simulink library "GOcontroll_Moduline_Target"  (R2023b)
settings: Solver=ode45  StartTime=0.0  StopTime=10.0  RelTol=1e-3  EnableMultiTasking=on
PreLoadFcn:
  | compile_gocontroll_mex;
values from neighbouring files (symbols this model uses):
  id = 2    [sfcn_UDPReceive.m]    (also in sfcn_UDPSend.m = 4)
undefined symbols (not defined in the file or in its folder): C_Cb1Pt10, Cb1Pt10_RAW_ERR_HIGH, Cb1Pt10_RAW_ERR_LOW, Cb1Pt10_SIG_ERR_HIGH, Cb1Pt10_SIG_ERR_LOW, Cb1Pt10_SIG_WAR_HIGH, Cb1Pt10_SIG_WAR_LOW, Pres_0_20_bar_500_4500_mv_inv, signal_x_RAW_ERR_HIGH, signal_x_RAW_ERR_LOW, signal_x_SIG_ERR_HIGH, signal_x_SIG_ERR_LOW, signal_x_SIG_WAR_HIGH, signal_x_SIG_WAR_LOW, signal_x_SPN, Valve1_ACTIVE_DUTY_CYCLE, Valve1_MAX_CURRENT, Valve1_MIN_CURRENT, Valve1_SPN
libraries: $bdroot x17, simulink x12, canmsglib x4
(part 5 of 5)

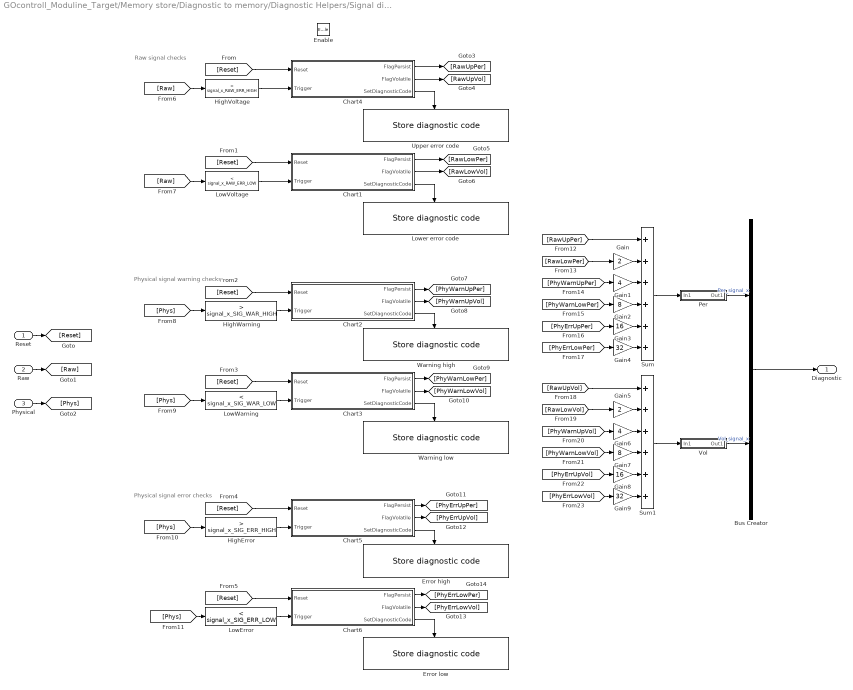
== system GOcontroll_Moduline_Target/Memory store/Diagnostic to memory/Diagnostic Helpers/Signal diagnostic ==
  note: Physical signal warning checks
  note: Raw signal checks
  note: Physical signal error checks
  Reset : Inport
  Raw : Inport  Port=2
  Physical : Inport  Port=3
  Enable : EnablePort
  Bus Creator : BusCreator  Inputs=2
  Chart1 : Stateflow chart  TreatAsAtomicUnit=on
  Chart2 : Stateflow chart  TreatAsAtomicUnit=on
  Chart3 : Stateflow chart  TreatAsAtomicUnit=on
  Chart4 : Stateflow chart  TreatAsAtomicUnit=on
  Chart5 : Stateflow chart  TreatAsAtomicUnit=on
  Chart6 : Stateflow chart  TreatAsAtomicUnit=on
  Error high : $bdroot/Memory store/Diagnostic to memory/Store diagnostic code  Tag=HANcoder_GOcontroll_Moduline_IV  spn=spn  fmi=(0) Data valid but above normal operational range, most severe level (3)  TriggerType=rising
  Error low : $bdroot/Memory store/Diagnostic to memory/Store diagnostic code  Tag=HANcoder_GOcontroll_Moduline_IV  spn=spn  fmi=(1) Data valid but below normal operational range, most severe level (3)  TriggerType=rising
  Gain : Gain  Gain=2
  Gain1 : Gain  Gain=4
  Gain2 : Gain  Gain=8
  Gain3 : Gain  Gain=16
  Gain4 : Gain  Gain=32
  Gain5 : Gain  Gain=2
  Gain6 : Gain  Gain=4
  Gain7 : Gain  Gain=8
  Gain8 : Gain  Gain=16
  Gain9 : Gain  Gain=32
  HighError : simulink/Logic and Bit Operations/Compare To Constant  relop=>  const=signal_x_SIG_ERR_HIGH  OutDataTypeStr=boolean
  HighVoltage : simulink/Logic and Bit Operations/Compare To Constant  relop=>  const=signal_x_RAW_ERR_HIGH  OutDataTypeStr=boolean
  HighWarning : simulink/Logic and Bit Operations/Compare To Constant  relop=>  const=signal_x_SIG_WAR_HIGH  OutDataTypeStr=boolean
  LowError : simulink/Logic and Bit Operations/Compare To Constant  relop=<  const=signal_x_SIG_ERR_LOW  OutDataTypeStr=boolean
  LowVoltage : simulink/Logic and Bit Operations/Compare To Constant  relop=<  const=signal_x_RAW_ERR_LOW  OutDataTypeStr=boolean
  LowWarning : simulink/Logic and Bit Operations/Compare To Constant  relop=<  const=signal_x_SIG_WAR_LOW  OutDataTypeStr=boolean
  Lower error code : $bdroot/Memory store/Diagnostic to memory/Store diagnostic code  Tag=HANcoder_GOcontroll_Moduline_IV  spn=spn  fmi=(4) Voltage below normal, or shorted to low source  TriggerType=rising
  Per : Subsystem
  Sum : Sum  Inputs=++++++  OutDataTypeStr=uint8
  Sum1 : Sum  Inputs=++++++  OutDataTypeStr=uint8
  Upper error code : $bdroot/Memory store/Diagnostic to memory/Store diagnostic code  Tag=HANcoder_GOcontroll_Moduline_IV  spn=spn  fmi=(3) Voltage above normal, or shorted to high source  TriggerType=rising
  Vol : Subsystem
  Warning high : $bdroot/Memory store/Diagnostic to memory/Store diagnostic code  Tag=HANcoder_GOcontroll_Moduline_IV  spn=spn  fmi=(15) Data valid but above normal range: least severe level (1)  TriggerType=rising
  Warning low : $bdroot/Memory store/Diagnostic to memory/Store diagnostic code  Tag=HANcoder_GOcontroll_Moduline_IV  spn=spn  fmi=(17) Data valid but below normal range: least severe level (1)  TriggerType=rising
  Diagnostic : Outport  OutputWhenDisabled=reset  InitialOutput=[0]
  wires:
  Chart4/3(SetDiagnosticCode) -> Upper error code/Trigger
  HighVoltage/1 -> Chart4/2(Trigger)
  LowVoltage/1 -> Chart1/2(Trigger)
  Chart1/3(SetDiagnosticCode) -> Lower error code/Trigger
  HighWarning/1 -> Chart2/2(Trigger)
  Chart2/3(SetDiagnosticCode) -> Warning high/Trigger
  LowWarning/1 -> Chart3/2(Trigger)
  Chart3/3(SetDiagnosticCode) -> Warning low/Trigger
  Chart6/3(SetDiagnosticCode) -> Error low/Trigger
  Chart5/3(SetDiagnosticCode) -> Error high/Trigger
  HighError/1 -> Chart5/2(Trigger)
  LowError/1 -> Chart6/2(Trigger)
  Reset/1 -> [Reset]
  [Reset] -> Chart4/1(Reset)
  [Reset] -> Chart1/1(Reset)
  [Reset] -> Chart2/1(Reset)
  [Reset] -> Chart3/1(Reset)
  [Reset] -> Chart5/1(Reset)
  [Reset] -> Chart6/1(Reset)
  Raw/1 -> [Raw]
  [Raw] -> HighVoltage/1
  [Raw] -> LowVoltage/1
  Physical/1 -> [Phys]
  [Phys] -> HighWarning/1
  [Phys] -> LowWarning/1
  [Phys] -> HighError/1
  [Phys] -> LowError/1
  Chart4/1(FlagPersist) -> [RawUpPer]
  Chart4/2(FlagVolatile) -> [RawUpVol]
  Chart1/1(FlagPersist) -> [RawLowPer]
  Chart1/2(FlagVolatile) -> [RawLowVol]
  Chart2/1(FlagPersist) -> [PhyWarnUpPer]
  Chart2/2(FlagVolatile) -> [PhyWarnUpVol]
  Chart3/1(FlagPersist) -> [PhyWarnLowPer]
  Chart3/2(FlagVolatile) -> [PhyWarnLowVol]
  Chart5/1(FlagPersist) -> [PhyErrUpPer]
  Chart5/2(FlagVolatile) -> [PhyErrUpVol]
  Chart6/1(FlagPersist) -> [PhyErrLowPer]
  Chart6/2(FlagVolatile) -> [PhyErrLowVol]
  [RawUpPer] -> Sum/1
  [RawLowPer] -> Gain/1
  Gain/1 -> Sum/2
  Gain1/1 -> Sum/3
  Gain4/1 -> Sum/6
  Gain3/1 -> Sum/5
  Gain2/1 -> Sum/4
  [PhyWarnUpPer] -> Gain1/1
  [PhyWarnLowPer] -> Gain2/1
  [PhyErrUpPer] -> Gain3/1
  [PhyErrLowPer] -> Gain4/1
  Sum/1 -> Per/1(In1)
  [RawUpVol] -> Sum1/1
  Gain9/1 -> Sum1/6
  Sum1/1 -> Vol/1(In1)
  Gain6/1 -> Sum1/3
  Gain5/1 -> Sum1/2
  Gain7/1 -> Sum1/4
  Gain8/1 -> Sum1/5
  [RawLowVol] -> Gain5/1
  [PhyWarnLowVol] -> Gain7/1
  [PhyWarnUpVol] -> Gain6/1
  [PhyErrUpVol] -> Gain8/1
  [PhyErrLowVol] -> Gain9/1
  Bus Creator/1 -> Diagnostic/1
  Vol/1(Out1) -> Bus Creator/2  "Vol_signal_x"
  Per/1(Out1) -> Bus Creator/1  "Per_signal_x"

== system GOcontroll_Moduline_Target/Network/UDP/UDP Example/Decode ==
  message : Inport
  message length : Inport  Port=2
  function : TriggerPort  TriggerType=function-call  VariantControl=(inherit)
  Compare To Constant : simulink/Logic and Bit Operations/Compare To Constant  relop===  const=5  OutDataTypeStr=boolean
  message len ok : Subsystem
  wires:
  message/1 -> message len ok/1(In1)
  message length/1 -> Compare To Constant/1
  Compare To Constant/1 -> message len ok/Enable

== system GOcontroll_Moduline_Target/Memory store/Diagnostic to memory/Diagnostic Helpers/Actuator diagnostic/Per ==
  In1 : Inport
  Out1 : Outport
  wires:
  In1/1 -> Out1/1

== system GOcontroll_Moduline_Target/Memory store/Diagnostic to memory/Diagnostic Helpers/Actuator diagnostic/Vol ==
  In1 : Inport
  Out1 : Outport
  wires:
  In1/1 -> Out1/1

== system GOcontroll_Moduline_Target/Memory store/Diagnostic to memory/Diagnostic Helpers/Signal diagnostic/Per ==
  In1 : Inport
  Out1 : Outport
  wires:
  In1/1 -> Out1/1

== system GOcontroll_Moduline_Target/Memory store/Diagnostic to memory/Diagnostic Helpers/Signal diagnostic/Vol ==
  In1 : Inport
  Out1 : Outport
  wires:
  In1/1 -> Out1/1

== system GOcontroll_Moduline_Target/Network/UDP/UDP Example/Decode/message len ok ==
  note: extract the data from bytes 1-4
  note: Check that the message ID in byte0 matches
  In1 : Inport
  Enable : EnablePort
  Compare To Constant1 : simulink/Logic and Bit Operations/Compare To Constant  relop===  const=0  OutDataTypeStr=boolean
  Selector : Selector  IndexMode=Zero-based  InputPortWidth=5  IndexOptions=Index vector (dialog)  Indices=[0]  OutputSizes=1
  Selector1 : Selector  IndexMode=Zero-based  InputPortWidth=5  IndexOptions=Starting index (dialog)  Indices=[1]  OutputSizes=4
  message id ok : Subsystem
  wires:
  Selector1/1 -> message id ok/1(In1)
  Selector/1 -> Compare To Constant1/1
  Compare To Constant1/1 -> message id ok/Enable
  In1/1 -> Selector/1, Selector1/1

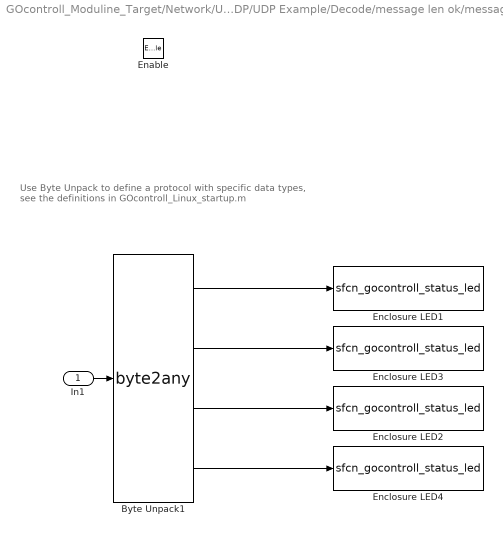
== system GOcontroll_Moduline_Target/Network/UDP/UDP Example/Decode/message len ok/message id ok ==
  note: Use Byte Unpack to define a protocol with
      | specific data types, see the definitions in
      | GOcontroll_Linux_startup.m
  In1 : Inport
  Enable : EnablePort
  Byte Unpack1 : S-Function  AncestorBlock=etargetslib/Byte Unpack  FunctionName=byte2any  Parameters=dimensionsout, datatypesout, byteAlign  SFunctionDeploymentMode=off  EnableBusSupport=off  mask(Byte Unpack){dimensions={1,1,1,1};, datatypes={'uint8','uint8','uint8','uint8'}, byteAlign=1}
      mask prompts: dimensions "Output port dimensions (cell array):"; datatypes "Output port data types (cell array):"; byteAlign "Byte alignment:"
      mask help: Unpack a binary byte vector to extract data. Insert after a UDP Recv block to break-up a UDP packet into its constituent data vectors.
      mask init:
      | [dimensionsout, datatypesout]= byteunpack_callback(dimensions, datatypes);
      mask Help: eval('linkfoundation.util.openBlockHelp(''etargetslibbyteunpack'')');
      mask TypeOptions byteAlign: 1 | 2 | 4 | 8
      mask Display:
      | color('blue');
      | text(0.95, 0.90, '', ...
      |                 'horizontalalignment', 'right');
      | color('black');
      | text(0.50, 0.12, 'Byte Unpack', ...
      |                 'horizontalAlignment','center');
  Enclosure LED1 : M-S-Function  Tag=HANcoder_TARGET_STM32_Olimexino  AncestorBlock=GOcontroll_Moduline_Target/Enclosure LED's/Enclosure LED  FunctionName=sfcn_gocontroll_status_led  Parameters=tsamp  mask(Enclosure LED's){tsamp=-1, led=1, color=Blue}
      mask prompts: tsamp "Sample time"
      mask help:
      | The Moduline controller is equipped with 4 RGB status LED's. To control them, simply configure the mask ( LED and color) and control them using uint8 values.
      |
      | Note: Moduline IV HW >= 3.02 has duty cycle controlled LED's. The intensity can be set from 0 (0%) to 255 (100%).
      |
      | LED: Select the LED that is needs to be controlled.
      |
      | Color: Select the color the LED needs to illuminate.
      mask init: same as GOcontroll_Moduline_Target/Enclosure LED's/Enclosure LED
      mask TypeOptions led: 1 | 2 | 3 | 4
      mask TypeOptions color: Red | Green | Blue
      mask Display:
      | fprintf('Status LED %d\nColor: %s',led,colorInfoStr);
      | text(2, 6, ert_linux_target_version());
  Enclosure LED2 : M-S-Function  Tag=HANcoder_TARGET_STM32_Olimexino  AncestorBlock=GOcontroll_Moduline_Target/Enclosure LED's/Enclosure LED  FunctionName=sfcn_gocontroll_status_led  Parameters=tsamp  mask(Enclosure LED's){tsamp=-1, led=3, color=Blue}
      mask prompts: tsamp "Sample time"
      mask help:
      | The Moduline controller is equipped with 4 RGB status LED's. To control them, simply configure the mask ( LED and color) and control them using uint8 values.
      |
      | Note: Moduline IV HW >= 3.02 has duty cycle controlled LED's. The intensity can be set from 0 (0%) to 255 (100%).
      |
      | LED: Select the LED that is needs to be controlled.
      |
      | Color: Select the color the LED needs to illuminate.
      mask init: same as GOcontroll_Moduline_Target/Enclosure LED's/Enclosure LED
      mask TypeOptions led: 1 | 2 | 3 | 4
      mask TypeOptions color: Red | Green | Blue
      mask Display:
      | fprintf('Status LED %d\nColor: %s',led,colorInfoStr);
      | text(2, 6, ert_linux_target_version());
  Enclosure LED3 : M-S-Function  Tag=HANcoder_TARGET_STM32_Olimexino  AncestorBlock=GOcontroll_Moduline_Target/Network/UDP/UDP Example/Decode/message len ok/message id ok/Enclosure LED2  FunctionName=sfcn_gocontroll_status_led  Parameters=tsamp  mask(Enclosure LED's){tsamp=-1, led=2, color=Blue}
      mask prompts: tsamp "Sample time"
      mask help:
      | The Moduline controller is equipped with 4 RGB status LED's. To control them, simply configure the mask ( LED and color) and control them using uint8 values.
      |
      | Note: Moduline IV HW >= 3.02 has duty cycle controlled LED's. The intensity can be set from 0 (0%) to 255 (100%).
      |
      | LED: Select the LED that is needs to be controlled.
      |
      | Color: Select the color the LED needs to illuminate.
      mask init: same as GOcontroll_Moduline_Target/Enclosure LED's/Enclosure LED
      mask TypeOptions led: 1 | 2 | 3 | 4
      mask TypeOptions color: Red | Green | Blue
      mask Display:
      | fprintf('Status LED %d\nColor: %s',led,colorInfoStr);
      | text(2, 6, ert_linux_target_version());
  Enclosure LED4 : M-S-Function  Tag=HANcoder_TARGET_STM32_Olimexino  AncestorBlock=GOcontroll_Moduline_Target/Network/UDP/UDP Example/Decode/message len ok/message id ok/Enclosure LED3  FunctionName=sfcn_gocontroll_status_led  Parameters=tsamp  mask(Enclosure LED's){tsamp=-1, led=4, color=Blue}
      mask prompts: tsamp "Sample time"
      mask help:
      | The Moduline controller is equipped with 4 RGB status LED's. To control them, simply configure the mask ( LED and color) and control them using uint8 values.
      |
      | Note: Moduline IV HW >= 3.02 has duty cycle controlled LED's. The intensity can be set from 0 (0%) to 255 (100%).
      |
      | LED: Select the LED that is needs to be controlled.
      |
      | Color: Select the color the LED needs to illuminate.
      mask init: same as GOcontroll_Moduline_Target/Enclosure LED's/Enclosure LED
      mask TypeOptions led: 1 | 2 | 3 | 4
      mask TypeOptions color: Red | Green | Blue
      mask Display:
      | fprintf('Status LED %d\nColor: %s',led,colorInfoStr);
      | text(2, 6, ert_linux_target_version());
  wires:
  In1/1 -> Byte Unpack1/1
  Byte Unpack1/2 -> Enclosure LED3/1
  Byte Unpack1/1 -> Enclosure LED1/1
  Byte Unpack1/3 -> Enclosure LED2/1
  Byte Unpack1/4 -> Enclosure LED4/1

== stateflow chart GOcontroll_Moduline_Target/Memory store/Diagnostic to memory/Diagnostic Helpers/Signal diagnostic/Chart2 ==
  state Entry
    en:SetDiagnosticCode = 0;
    en:FlagPersist = 0;
    en:FlagVolatile = 0;
  state Reset_Flag
    state System_Running
      en:FlagVolatile = 0;
    state Error_Triggered
    state Error_Triggered_Confirmed
      en:SetDiagnosticCode = 1;
      en:FlagPersist = 1;
      en:FlagVolatile = 1;
    state Error_Code_Stored
      en:SetDiagnosticCode = 0;
    System_Running -> Error_Triggered : [Trigger == 1]
    Error_Triggered -> System_Running [order 2] : [Trigger == 0]
    Error_Code_Stored -> System_Running : [Trigger == 0]
    Error_Triggered -> Error_Triggered_Confirmed [order 1] : [after(duration,msec)]
    Error_Triggered_Confirmed -> Error_Code_Stored : [after(1,sec)]
  (default) -> Entry
  Entry -> System_Running : [after(delay,msec)]
  Reset_Flag -> Entry : [Reset == 1]
  data: Reset input; FlagPersist output; FlagVolatile output; Trigger input; SetDiagnosticCode output uint8; delay parameter single; duration parameter single

== stateflow chart GOcontroll_Moduline_Target/Memory store/Diagnostic to memory/Diagnostic Helpers/Signal diagnostic/Chart3 ==
  state Entry
    en:SetDiagnosticCode = 0;
    en:FlagPersist = 0;
    en:FlagVolatile = 0;
  state Reset_Flag
    state System_Running
      en:FlagVolatile = 0;
    state Error_Triggered
    state Error_Triggered_Confirmed
      en:SetDiagnosticCode = 1;
      en:FlagPersist = 1;
      en:FlagVolatile = 1;
    state Error_Code_Stored
      en:SetDiagnosticCode = 0;
    System_Running -> Error_Triggered : [Trigger == 1]
    Error_Triggered -> System_Running [order 2] : [Trigger == 0]
    Error_Code_Stored -> System_Running : [Trigger == 0]
    Error_Triggered -> Error_Triggered_Confirmed [order 1] : [after(duration,msec)]
    Error_Triggered_Confirmed -> Error_Code_Stored : [after(1,sec)]
  (default) -> Entry
  Entry -> System_Running : [after(delay,msec)]
  Reset_Flag -> Entry : [Reset == 1]
  data: Reset input; FlagPersist output; FlagVolatile output; Trigger input; SetDiagnosticCode output uint8; delay parameter single; duration parameter single

== stateflow chart GOcontroll_Moduline_Target/Memory store/Diagnostic to memory/Diagnostic Helpers/Signal diagnostic/Chart4 ==
  state Entry
    en:SetDiagnosticCode = 0;
    en:FlagPersist = 0;
    en:FlagVolatile = 0;
  state Reset_Flag
    state System_Running
      en:FlagVolatile = 0;
    state Error_Triggered
    state Error_Triggered_Confirmed
      en:SetDiagnosticCode = 1;
      en:FlagPersist = 1;
      en:FlagVolatile = 1;
    state Error_Code_Stored
      en:SetDiagnosticCode = 0;
    System_Running -> Error_Triggered : [Trigger == 1]
    Error_Triggered -> System_Running [order 2] : [Trigger == 0]
    Error_Code_Stored -> System_Running : [Trigger == 0]
    Error_Triggered -> Error_Triggered_Confirmed [order 1] : [after(duration,msec)]
    Error_Triggered_Confirmed -> Error_Code_Stored : [after(1,sec)]
  (default) -> Entry
  Entry -> System_Running : [after(delay,msec)]
  Reset_Flag -> Entry : [Reset == 1]
  data: Reset input; FlagPersist output; FlagVolatile output; Trigger input; SetDiagnosticCode output uint8; delay parameter single; duration parameter single

== stateflow chart GOcontroll_Moduline_Target/Memory store/Diagnostic to memory/Diagnostic Helpers/Signal diagnostic/Chart5 ==
  state Entry
    en:SetDiagnosticCode = 0;
    en:FlagPersist = 0;
    en:FlagVolatile = 0;
  state Reset_Flag
    state System_Running
      en:FlagVolatile = 0;
    state Error_Triggered
    state Error_Triggered_Confirmed
      en:SetDiagnosticCode = 1;
      en:FlagPersist = 1;
      en:FlagVolatile = 1;
    state Error_Code_Stored
      en:SetDiagnosticCode = 0;
    System_Running -> Error_Triggered : [Trigger == 1]
    Error_Triggered -> System_Running [order 2] : [Trigger == 0]
    Error_Code_Stored -> System_Running : [Trigger == 0]
    Error_Triggered -> Error_Triggered_Confirmed [order 1] : [after(duration,msec)]
    Error_Triggered_Confirmed -> Error_Code_Stored : [after(1,sec)]
  (default) -> Entry
  Entry -> System_Running : [after(delay,msec)]
  Reset_Flag -> Entry : [Reset == 1]
  data: Reset input; FlagPersist output; FlagVolatile output; Trigger input; SetDiagnosticCode output uint8; delay parameter single; duration parameter single

== stateflow chart GOcontroll_Moduline_Target/Memory store/Diagnostic to memory/Diagnostic Helpers/Signal diagnostic/Chart6 ==
  state Entry
    en:SetDiagnosticCode = 0;
    en:FlagPersist = 0;
    en:FlagVolatile = 0;
  state Reset_Flag
    state System_Running
      en:FlagVolatile = 0;
    state Error_Triggered
    state Error_Triggered_Confirmed
      en:SetDiagnosticCode = 1;
      en:FlagPersist = 1;
      en:FlagVolatile = 1;
    state Error_Code_Stored
      en:SetDiagnosticCode = 0;
    System_Running -> Error_Triggered : [Trigger == 1]
    Error_Triggered -> System_Running [order 2] : [Trigger == 0]
    Error_Code_Stored -> System_Running : [Trigger == 0]
    Error_Triggered -> Error_Triggered_Confirmed [order 1] : [after(duration,msec)]
    Error_Triggered_Confirmed -> Error_Code_Stored : [after(1,sec)]
  (default) -> Entry
  Entry -> System_Running : [after(delay,msec)]
  Reset_Flag -> Entry : [Reset == 1]
  data: Reset input; FlagPersist output; FlagVolatile output; Trigger input; SetDiagnosticCode output uint8; delay parameter single; duration parameter single

== stateflow chart GOcontroll_Moduline_Target/Memory store/Diagnostic to memory/Diagnostic Helpers/Actuator diagnostic/Chart1 ==
  state Entry
    en:SetDiagnosticCode = 0;
    en:FlagPersist = uint8(0);
    en:FlagVolatile = uint8(0);
  state Reset_Flag
    state System_Running
      en:FlagVolatile = 0;
    state Error_Triggered
    state Error_Triggered_Confirmed
      en:SetDiagnosticCode = 1;
      en:FlagPersist = 1;
      en:FlagVolatile = 1;
    state Error_Code_Stored
      en:SetDiagnosticCode = 0;
    System_Running -> Error_Triggered : [Trigger == 1]
    Error_Triggered -> System_Running [order 2] : [Trigger == 0]
    Error_Code_Stored -> System_Running : [Trigger == 0]
    Error_Triggered -> Error_Triggered_Confirmed [order 1] : [after(duration,msec)]
    Error_Triggered_Confirmed -> Error_Code_Stored : [after(1,sec)]
  (default) -> Entry
  Entry -> System_Running : [after(delay,msec)]
  Reset_Flag -> Entry : [Reset == 1]
  data: Reset input; FlagPersist output; FlagVolatile output; Trigger input; SetDiagnosticCode output uint8; delay parameter single; duration parameter single

== stateflow chart GOcontroll_Moduline_Target/Memory store/Diagnostic to memory/Diagnostic Helpers/Actuator diagnostic/Chart4 ==
  state Entry
    en:SetDiagnosticCode = 0;
    en:FlagPersist = uint8(0);
    en:FlagVolatile = uint8(0);
  state Reset_Flag
    state System_Running
      en:FlagVolatile = 0;
    state Error_Triggered
    state Error_Triggered_Confirmed
      en:SetDiagnosticCode = 1;
      en:FlagPersist = 1;
      en:FlagVolatile = 1;
    state Error_Code_Stored
      en:SetDiagnosticCode = 0;
    System_Running -> Error_Triggered : [Trigger == 1]
    Error_Triggered -> System_Running [order 2] : [Trigger == 0]
    Error_Code_Stored -> System_Running : [Trigger == 0]
    Error_Triggered -> Error_Triggered_Confirmed [order 1] : [after(duration,msec)]
    Error_Triggered_Confirmed -> Error_Code_Stored : [after(1,sec)]
  (default) -> Entry
  Entry -> System_Running : [after(delay,msec)]
  Reset_Flag -> Entry : [Reset == 1]
  data: Reset input; FlagPersist output; FlagVolatile output; Trigger input; SetDiagnosticCode output uint8; delay parameter single; duration parameter single

== stateflow chart GOcontroll_Moduline_Target/Memory store/Diagnostic to memory/Diagnostic Helpers/Generic diagnostic/Chart4 ==
  state Entry
    en:SetDiagnosticCode = 0;
    en:FlagPersist = uint8(0);
    en:FlagVolatile = uint8(0);
  state Reset_Flag
    state System_Running
      en:FlagVolatile = 0;
    state Error_Triggered
    state Error_Triggered_Confirmed
      en:SetDiagnosticCode = 1;
      en:FlagPersist = 1;
      en:FlagVolatile = 1;
    state Error_Code_Stored
      en:SetDiagnosticCode = 0;
    System_Running -> Error_Triggered : [Trigger == 1]
    Error_Triggered -> System_Running [order 2] : [Trigger == 0]
    Error_Code_Stored -> System_Running : [Trigger == 0]
    Error_Triggered -> Error_Triggered_Confirmed [order 1] : [after(duration,msec)]
    Error_Triggered_Confirmed -> Error_Code_Stored : [after(1,sec)]
  (default) -> Entry
  Entry -> System_Running : [after(delay,msec)]
  Reset_Flag -> Entry : [Reset == 1]
  data: Reset input; FlagPersist output; FlagVolatile output; Trigger input; SetDiagnosticCode output uint8; delay parameter single; duration parameter single

== stateflow chart GOcontroll_Moduline_Target/Memory store/Diagnostic to memory/Diagnostic Helpers/Signal diagnostic/Chart1 ==
  state Entry
    en:SetDiagnosticCode = 0;
    en:FlagPersist = 0;
    en:FlagVolatile = 0;
  state Reset_Flag
    state System_Running
      en:FlagVolatile = 0;
    state Error_Triggered
    state Error_Triggered_Confirmed
      en:SetDiagnosticCode = 1;
      en:FlagPersist = 1;
      en:FlagVolatile = 1;
    state Error_Code_Stored
      en:SetDiagnosticCode = 0;
    System_Running -> Error_Triggered : [Trigger == 1]
    Error_Triggered -> System_Running [order 2] : [Trigger == 0]
    Error_Code_Stored -> System_Running : [Trigger == 0]
    Error_Triggered -> Error_Triggered_Confirmed [order 1] : [after(duration,msec)]
    Error_Triggered_Confirmed -> Error_Code_Stored : [after(1,sec)]
  (default) -> Entry
  Entry -> System_Running : [after(delay,msec)]
  Reset_Flag -> Entry : [Reset == 1]
  data: Reset input; FlagPersist output; FlagVolatile output; Trigger input; SetDiagnosticCode output uint8; delay parameter single; duration parameter single
